simulink model "full_order_with_resistances_to_pdf"  (R2015b)
settings: Solver=VariableStepAuto  StartTime=0.0  StopTime=10.0  RelTol=1e-3
undefined symbols (not defined in the file): C, J, Kt, Kv, L, R, TL, Vin
settings Model: Creator=Morten  LastModifiedBy=Morten

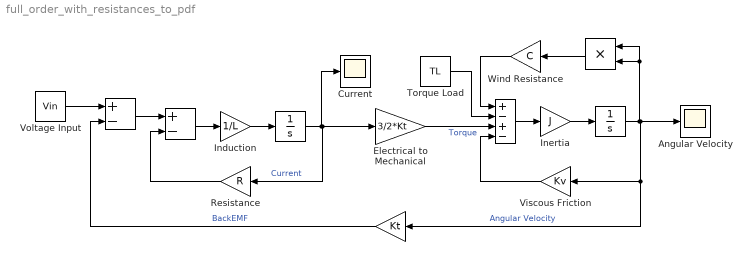
== system full_order_with_resistances_to_pdf ==
  "  " : Sum  Inputs=+-
  "   " : Sum  Inputs=+-
  "    " : Sum  Inputs=+-+-
  "          " : Product
  "                          " : Integrator
  "                            " : Gain  Gain=Kt
  "                                     " : Integrator
  Angular Velocity : Scope
  Current : Scope
  Electrical to Mechanical : Gain  Gain=3/2*Kt
  Induction : Gain  Gain=1/L
  Inertia : Gain  Gain=J
  Resistance : Gain  Gain=R
  Torque Load : Constant  Value=TL
  Viscous Friction : Gain  Gain=Kv
  Voltage Input : Constant  Value=Vin
  Wind Resistance : Gain  Gain=C
  wires:
  "    "/1 -> Inertia/1
  "                          "/1 -> Current/1, Resistance/1, Electrical to Mechanical/1  "Current"
  Resistance/1 -> "   "/2
  "                            "/1 -> "  "/2  "BackEMF"
  Inertia/1 -> "                                     "/1
  "  "/1 -> "   "/1
  "   "/1 -> Induction/1
  Induction/1 -> "                          "/1
  Voltage Input/1 -> "  "/1
  "          "/1 -> Wind Resistance/1
  Wind Resistance/1 -> "    "/1
  "                                     "/1 -> Angular Velocity/1, "                            "/1, Viscous Friction/1, "          "/2, "          "/1  "Angular Velocity"
  Electrical to Mechanical/1 -> "    "/3  "Torque"
  Viscous Friction/1 -> "    "/4
  Torque Load/1 -> "    "/2
